simulink model "eci2tle_test"  (R2016b)
settings: Solver=VariableStepAuto  StartTime=0.0  StopTime=0  RelTol=1e-3
undefined symbols (not defined in the file or in its folder): fsw_params
libraries: gps x1, GPS_processing_lib x1, GPS_time_lib x1, time_coord_rotation_lib x1, tle2eci_coarse_lib x1
settings Model: Creator=Taylor  LastModifiedBy=taylorreynolds

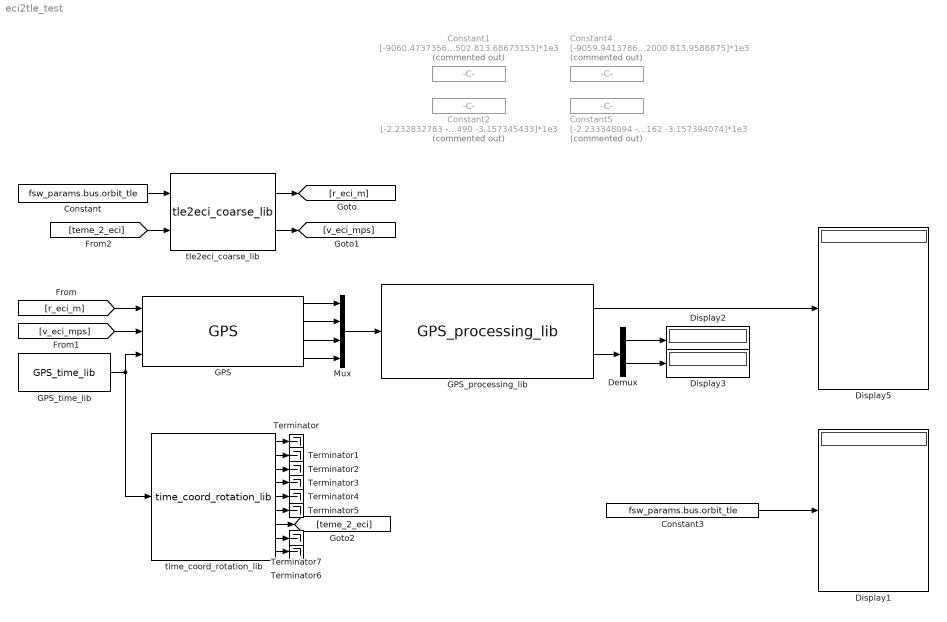
== system eci2tle_test ==
  Constant : Constant  Value=fsw_params.bus.orbit_tle
  Constant1 : Constant  Commented=on  Value=[-9060.47373569 4658.70952502 813.68673153]*1e3
  Constant2 : Constant  Commented=on  Value=[-2.232832783 -4.110453490 -3.157345433]*1e3
  Constant3 : Constant  Value=fsw_params.bus.orbit_tle
  Constant4 : Constant  Commented=on  Value=[-9059.9413786 4659.6972000 813.9588875]*1e3
  Constant5 : Constant  Commented=on  Value=[-2.233348094 -4.110136162 -3.157394074]*1e3
  Demux : Demux  Outputs=2
  Display{1..3,5} (4 alike) : Display
  GPS : gps/GPS
  GPS_processing_lib : GPS_processing_lib/GPS_processing_lib
  GPS_time_lib : GPS_time_lib/GPS_time_lib
  Mux : Mux  Inputs=[3 3 2 1]
  Terminator{,1..7} (8 alike) : Terminator
  time_coord_rotation_lib : time_coord_rotation_lib/time_coord_rotation_lib
  tle2eci_coarse_lib : tle2eci_coarse_lib/tle2eci_coarse_lib
  wires:
  Constant3/1 -> Display1/1
  Mux/1 -> GPS_processing_lib/1
  GPS/1 -> Mux/1
  GPS/2 -> Mux/2
  GPS/3 -> Mux/3
  GPS/4 -> Mux/4
  Constant/1 -> tle2eci_coarse_lib/1
  tle2eci_coarse_lib/1 -> [r_eci_m]
  tle2eci_coarse_lib/2 -> [v_eci_mps]
  [r_eci_m] -> GPS/1
  [v_eci_mps] -> GPS/2
  GPS_processing_lib/2 -> Demux/1
  Demux/1 -> Display2/1
  Demux/2 -> Display3/1
  GPS_time_lib/1 -> time_coord_rotation_lib/1, GPS/3
  time_coord_rotation_lib/7 -> [teme_2_eci]
  [teme_2_eci] -> tle2eci_coarse_lib/2
  GPS_processing_lib/1 -> Display5/1
  time_coord_rotation_lib/1 -> Terminator/1
  time_coord_rotation_lib/2 -> Terminator1/1
  time_coord_rotation_lib/3 -> Terminator2/1
  time_coord_rotation_lib/4 -> Terminator3/1
  time_coord_rotation_lib/5 -> Terminator4/1
  time_coord_rotation_lib/6 -> Terminator5/1
  time_coord_rotation_lib/9 -> Terminator6/1
  time_coord_rotation_lib/8 -> Terminator7/1
